simulink model "Charge_2_V1_FreeCharge"  (R2018b)
settings: Solver=FixedStepDiscrete  StartTime=0.0  StopTime=1  FixedStep=0.001  RelTol=1e-3
PreLoadFcn:
  | librarySetup
  | eval([bdroot,'_startup']) %Calling [modelName]_startup.m
undefined symbols (not defined in the file or in its folder): A0, A1, Car1__Authorize, Car2_Authorize, CON2, CON3, CON4, Control_Mode_In, CurrentSP, D10, D12, D13, D2, D3, D4, D5, D6, D7, D8, Free_Charge, Frequency_High_Point, Frequency_Low_Point, Frequency_Mid_high, Frequency_Mid_low, HVol_High_Point, HVol_Low_Point, HVol_Mid_high, HVol_Mid_low, HVoltage_Factor, SeconCar_ThreePhase, V_Current_five, V_Current_four, V_Current_one, V_Current_six, V_Current_three, V_Current_two, V_Frequency, V_MaxPliot, V_MinPliot, Vol_High_Point, Vol_Low_Point, Vol_Mid_high, Vol_Mid_low, Voltage_Factor, Voltage_Mode_Test
libraries: simulink x331, HANcoder_STM32_Target x30, powerlib_meascontrol x8, simulink_extras x2
(part 7 of 13)

== system Charge_2_V1_FreeCharge/HANcoder STM32 Target - E407-STM32 algorithm/Energy Meter1/Energy_Meter_Recieve/Voltage_Meter_2/Read_Gyro12 ==
  Trigger : TriggerPort  VariantControl=Variant
  UART receive : Subsystem  AncestorBlock=HANcoder_STM32_Target/STM32-E407/UART/UART receive  mask(UART receive){channel=UART2: Con. PD-8 & Con. PD-9 (PD5 & PD6), useStatusOut=off, tsamp=-1}
      mask prompts: useStatusOut "Use status outport"; tsamp "Sample time"
      mask help:
      | Function
      | ==========
      | Reads a byte from the UART reception buffer.
      |
      | Parameters per channel
      | ======================
      | - Select channel
      | - Select if the status output should be enabled.
      |
      | Outputs
      | =======
      | - The value of the receive byte.
      | - When the status output is 0, the reception buffer was empty.
      mask init:
      | uartChannelInfoStr = sfcn_uart_receive_mcb(2, channel, useStatusOut);
      settings: MoveFcn=drawLogos
      mask Help: web('sfcn_uart_receive.html')
      mask TypeOptions channel: UART1: Con. 3-D1 & Con. 3-D0 (PB6 & PB7) | UART2: Con. PD-8 & Con. PD-9 (PD5 & PD6) | UART3: Con. PD-11 & Con. PD-12 (PD8 & PD9) | UART6: Con. UEXT-3 & Con. UEXT-4 (PC6 & PC7)
      mask Display: fprintf('UART receive\n%s', uartChannelInfoStr);patch([240 246 246],[8 14 2],[1 0 0]);patch([248 248 254],[14 2 8],[0 0 0.35]);
  Out1 : Outport
  wires:
  UART receive/1(Out1) -> Out1/1

== system Charge_2_V1_FreeCharge/HANcoder STM32 Target - E407-STM32 algorithm/Energy Meter1/Energy_Meter_Recieve/Voltage_Meter_2/Read_Gyro13 ==
  Trigger : TriggerPort  VariantControl=Variant
  UART receive : Subsystem  AncestorBlock=HANcoder_STM32_Target/STM32-E407/UART/UART receive  mask(UART receive){channel=UART2: Con. PD-8 & Con. PD-9 (PD5 & PD6), useStatusOut=off, tsamp=-1}
      mask prompts: useStatusOut "Use status outport"; tsamp "Sample time"
      mask help:
      | Function
      | ==========
      | Reads a byte from the UART reception buffer.
      |
      | Parameters per channel
      | ======================
      | - Select channel
      | - Select if the status output should be enabled.
      |
      | Outputs
      | =======
      | - The value of the receive byte.
      | - When the status output is 0, the reception buffer was empty.
      mask init:
      | uartChannelInfoStr = sfcn_uart_receive_mcb(2, channel, useStatusOut);
      settings: MoveFcn=drawLogos
      mask Help: web('sfcn_uart_receive.html')
      mask TypeOptions channel: UART1: Con. 3-D1 & Con. 3-D0 (PB6 & PB7) | UART2: Con. PD-8 & Con. PD-9 (PD5 & PD6) | UART3: Con. PD-11 & Con. PD-12 (PD8 & PD9) | UART6: Con. UEXT-3 & Con. UEXT-4 (PC6 & PC7)
      mask Display: fprintf('UART receive\n%s', uartChannelInfoStr);patch([240 246 246],[8 14 2],[1 0 0]);patch([248 248 254],[14 2 8],[0 0 0.35]);
  Out1 : Outport
  wires:
  UART receive/1(Out1) -> Out1/1

== system Charge_2_V1_FreeCharge/HANcoder STM32 Target - E407-STM32 algorithm/Energy Meter1/Energy_Meter_Recieve/Voltage_Meter_2/Read_Gyro14 ==
  Trigger : TriggerPort  VariantControl=Variant
  UART receive : Subsystem  AncestorBlock=HANcoder_STM32_Target/STM32-E407/UART/UART receive  mask(UART receive){channel=UART2: Con. PD-8 & Con. PD-9 (PD5 & PD6), useStatusOut=off, tsamp=-1}
      mask prompts: useStatusOut "Use status outport"; tsamp "Sample time"
      mask help:
      | Function
      | ==========
      | Reads a byte from the UART reception buffer.
      |
      | Parameters per channel
      | ======================
      | - Select channel
      | - Select if the status output should be enabled.
      |
      | Outputs
      | =======
      | - The value of the receive byte.
      | - When the status output is 0, the reception buffer was empty.
      mask init:
      | uartChannelInfoStr = sfcn_uart_receive_mcb(2, channel, useStatusOut);
      settings: MoveFcn=drawLogos
      mask Help: web('sfcn_uart_receive.html')
      mask TypeOptions channel: UART1: Con. 3-D1 & Con. 3-D0 (PB6 & PB7) | UART2: Con. PD-8 & Con. PD-9 (PD5 & PD6) | UART3: Con. PD-11 & Con. PD-12 (PD8 & PD9) | UART6: Con. UEXT-3 & Con. UEXT-4 (PC6 & PC7)
      mask Display: fprintf('UART receive\n%s', uartChannelInfoStr);patch([240 246 246],[8 14 2],[1 0 0]);patch([248 248 254],[14 2 8],[0 0 0.35]);
  Out1 : Outport
  wires:
  UART receive/1(Out1) -> Out1/1

== system Charge_2_V1_FreeCharge/HANcoder STM32 Target - E407-STM32 algorithm/Energy Meter1/Energy_Meter_Recieve/Voltage_Meter_2/Read_Gyro15 ==
  Trigger : TriggerPort  VariantControl=Variant
  UART receive : Subsystem  AncestorBlock=HANcoder_STM32_Target/STM32-E407/UART/UART receive  mask(UART receive){channel=UART2: Con. PD-8 & Con. PD-9 (PD5 & PD6), useStatusOut=off, tsamp=-1}
      mask prompts: useStatusOut "Use status outport"; tsamp "Sample time"
      mask help:
      | Function
      | ==========
      | Reads a byte from the UART reception buffer.
      |
      | Parameters per channel
      | ======================
      | - Select channel
      | - Select if the status output should be enabled.
      |
      | Outputs
      | =======
      | - The value of the receive byte.
      | - When the status output is 0, the reception buffer was empty.
      mask init:
      | uartChannelInfoStr = sfcn_uart_receive_mcb(2, channel, useStatusOut);
      settings: MoveFcn=drawLogos
      mask Help: web('sfcn_uart_receive.html')
      mask TypeOptions channel: UART1: Con. 3-D1 & Con. 3-D0 (PB6 & PB7) | UART2: Con. PD-8 & Con. PD-9 (PD5 & PD6) | UART3: Con. PD-11 & Con. PD-12 (PD8 & PD9) | UART6: Con. UEXT-3 & Con. UEXT-4 (PC6 & PC7)
      mask Display: fprintf('UART receive\n%s', uartChannelInfoStr);patch([240 246 246],[8 14 2],[1 0 0]);patch([248 248 254],[14 2 8],[0 0 0.35]);
  Out1 : Outport
  wires:
  UART receive/1(Out1) -> Out1/1

== system Charge_2_V1_FreeCharge/HANcoder STM32 Target - E407-STM32 algorithm/Energy Meter1/Energy_Meter_Recieve/Voltage_Meter_2/Read_Gyro16 ==
  Trigger : TriggerPort  VariantControl=Variant
  UART receive : Subsystem  AncestorBlock=HANcoder_STM32_Target/STM32-E407/UART/UART receive  mask(UART receive){channel=UART2: Con. PD-8 & Con. PD-9 (PD5 & PD6), useStatusOut=off, tsamp=-1}
      mask prompts: useStatusOut "Use status outport"; tsamp "Sample time"
      mask help:
      | Function
      | ==========
      | Reads a byte from the UART reception buffer.
      |
      | Parameters per channel
      | ======================
      | - Select channel
      | - Select if the status output should be enabled.
      |
      | Outputs
      | =======
      | - The value of the receive byte.
      | - When the status output is 0, the reception buffer was empty.
      mask init:
      | uartChannelInfoStr = sfcn_uart_receive_mcb(2, channel, useStatusOut);
      settings: MoveFcn=drawLogos
      mask Help: web('sfcn_uart_receive.html')
      mask TypeOptions channel: UART1: Con. 3-D1 & Con. 3-D0 (PB6 & PB7) | UART2: Con. PD-8 & Con. PD-9 (PD5 & PD6) | UART3: Con. PD-11 & Con. PD-12 (PD8 & PD9) | UART6: Con. UEXT-3 & Con. UEXT-4 (PC6 & PC7)
      mask Display: fprintf('UART receive\n%s', uartChannelInfoStr);patch([240 246 246],[8 14 2],[1 0 0]);patch([248 248 254],[14 2 8],[0 0 0.35]);
  Out1 : Outport
  wires:
  UART receive/1(Out1) -> Out1/1

== system Charge_2_V1_FreeCharge/HANcoder STM32 Target - E407-STM32 algorithm/Energy Meter1/Energy_Meter_Recieve/Voltage_Meter_2/Read_Gyro17 ==
  Trigger : TriggerPort  VariantControl=Variant
  UART receive : Subsystem  AncestorBlock=HANcoder_STM32_Target/STM32-E407/UART/UART receive  mask(UART receive){channel=UART2: Con. PD-8 & Con. PD-9 (PD5 & PD6), useStatusOut=off, tsamp=-1}
      mask prompts: useStatusOut "Use status outport"; tsamp "Sample time"
      mask help:
      | Function
      | ==========
      | Reads a byte from the UART reception buffer.
      |
      | Parameters per channel
      | ======================
      | - Select channel
      | - Select if the status output should be enabled.
      |
      | Outputs
      | =======
      | - The value of the receive byte.
      | - When the status output is 0, the reception buffer was empty.
      mask init:
      | uartChannelInfoStr = sfcn_uart_receive_mcb(2, channel, useStatusOut);
      settings: MoveFcn=drawLogos
      mask Help: web('sfcn_uart_receive.html')
      mask TypeOptions channel: UART1: Con. 3-D1 & Con. 3-D0 (PB6 & PB7) | UART2: Con. PD-8 & Con. PD-9 (PD5 & PD6) | UART3: Con. PD-11 & Con. PD-12 (PD8 & PD9) | UART6: Con. UEXT-3 & Con. UEXT-4 (PC6 & PC7)
      mask Display: fprintf('UART receive\n%s', uartChannelInfoStr);patch([240 246 246],[8 14 2],[1 0 0]);patch([248 248 254],[14 2 8],[0 0 0.35]);
  Out1 : Outport
  wires:
  UART receive/1(Out1) -> Out1/1

== system Charge_2_V1_FreeCharge/HANcoder STM32 Target - E407-STM32 algorithm/Energy Meter1/Energy_Meter_Recieve/Voltage_Meter_2/Read_Gyro18 ==
  Trigger : TriggerPort  VariantControl=Variant
  UART receive : Subsystem  AncestorBlock=HANcoder_STM32_Target/STM32-E407/UART/UART receive  mask(UART receive){channel=UART2: Con. PD-8 & Con. PD-9 (PD5 & PD6), useStatusOut=off, tsamp=-1}
      mask prompts: useStatusOut "Use status outport"; tsamp "Sample time"
      mask help:
      | Function
      | ==========
      | Reads a byte from the UART reception buffer.
      |
      | Parameters per channel
      | ======================
      | - Select channel
      | - Select if the status output should be enabled.
      |
      | Outputs
      | =======
      | - The value of the receive byte.
      | - When the status output is 0, the reception buffer was empty.
      mask init:
      | uartChannelInfoStr = sfcn_uart_receive_mcb(2, channel, useStatusOut);
      settings: MoveFcn=drawLogos
      mask Help: web('sfcn_uart_receive.html')
      mask TypeOptions channel: UART1: Con. 3-D1 & Con. 3-D0 (PB6 & PB7) | UART2: Con. PD-8 & Con. PD-9 (PD5 & PD6) | UART3: Con. PD-11 & Con. PD-12 (PD8 & PD9) | UART6: Con. UEXT-3 & Con. UEXT-4 (PC6 & PC7)
      mask Display: fprintf('UART receive\n%s', uartChannelInfoStr);patch([240 246 246],[8 14 2],[1 0 0]);patch([248 248 254],[14 2 8],[0 0 0.35]);
  Out1 : Outport
  wires:
  UART receive/1(Out1) -> Out1/1

== system Charge_2_V1_FreeCharge/HANcoder STM32 Target - E407-STM32 algorithm/Energy Meter1/Energy_Meter_Recieve/Voltage_Meter_2/Read_Gyro2 ==
  Trigger : TriggerPort  VariantControl=Variant
  UART receive : Subsystem  AncestorBlock=HANcoder_STM32_Target/STM32-E407/UART/UART receive  mask(UART receive){channel=UART2: Con. PD-8 & Con. PD-9 (PD5 & PD6), useStatusOut=off, tsamp=-1}
      mask prompts: useStatusOut "Use status outport"; tsamp "Sample time"
      mask help:
      | Function
      | ==========
      | Reads a byte from the UART reception buffer.
      |
      | Parameters per channel
      | ======================
      | - Select channel
      | - Select if the status output should be enabled.
      |
      | Outputs
      | =======
      | - The value of the receive byte.
      | - When the status output is 0, the reception buffer was empty.
      mask init:
      | uartChannelInfoStr = sfcn_uart_receive_mcb(2, channel, useStatusOut);
      settings: MoveFcn=drawLogos
      mask Help: web('sfcn_uart_receive.html')
      mask TypeOptions channel: UART1: Con. 3-D1 & Con. 3-D0 (PB6 & PB7) | UART2: Con. PD-8 & Con. PD-9 (PD5 & PD6) | UART3: Con. PD-11 & Con. PD-12 (PD8 & PD9) | UART6: Con. UEXT-3 & Con. UEXT-4 (PC6 & PC7)
      mask Display: fprintf('UART receive\n%s', uartChannelInfoStr);patch([240 246 246],[8 14 2],[1 0 0]);patch([248 248 254],[14 2 8],[0 0 0.35]);
  Out1 : Outport
  wires:
  UART receive/1(Out1) -> Out1/1

== system Charge_2_V1_FreeCharge/HANcoder STM32 Target - E407-STM32 algorithm/Energy Meter1/Energy_Meter_Recieve/Voltage_Meter_2/Read_Gyro3 ==
  Trigger : TriggerPort  VariantControl=Variant
  UART receive : Subsystem  AncestorBlock=HANcoder_STM32_Target/STM32-E407/UART/UART receive  mask(UART receive){channel=UART2: Con. PD-8 & Con. PD-9 (PD5 & PD6), useStatusOut=off, tsamp=-1}
      mask prompts: useStatusOut "Use status outport"; tsamp "Sample time"
      mask help:
      | Function
      | ==========
      | Reads a byte from the UART reception buffer.
      |
      | Parameters per channel
      | ======================
      | - Select channel
      | - Select if the status output should be enabled.
      |
      | Outputs
      | =======
      | - The value of the receive byte.
      | - When the status output is 0, the reception buffer was empty.
      mask init:
      | uartChannelInfoStr = sfcn_uart_receive_mcb(2, channel, useStatusOut);
      settings: MoveFcn=drawLogos
      mask Help: web('sfcn_uart_receive.html')
      mask TypeOptions channel: UART1: Con. 3-D1 & Con. 3-D0 (PB6 & PB7) | UART2: Con. PD-8 & Con. PD-9 (PD5 & PD6) | UART3: Con. PD-11 & Con. PD-12 (PD8 & PD9) | UART6: Con. UEXT-3 & Con. UEXT-4 (PC6 & PC7)
      mask Display: fprintf('UART receive\n%s', uartChannelInfoStr);patch([240 246 246],[8 14 2],[1 0 0]);patch([248 248 254],[14 2 8],[0 0 0.35]);
  Out1 : Outport
  wires:
  UART receive/1(Out1) -> Out1/1

== system Charge_2_V1_FreeCharge/HANcoder STM32 Target - E407-STM32 algorithm/Energy Meter1/Energy_Meter_Recieve/Voltage_Meter_2/Read_Gyro4 ==
  Trigger : TriggerPort  VariantControl=Variant
  UART receive : Subsystem  AncestorBlock=HANcoder_STM32_Target/STM32-E407/UART/UART receive  mask(UART receive){channel=UART2: Con. PD-8 & Con. PD-9 (PD5 & PD6), useStatusOut=off, tsamp=-1}
      mask prompts: useStatusOut "Use status outport"; tsamp "Sample time"
      mask help:
      | Function
      | ==========
      | Reads a byte from the UART reception buffer.
      |
      | Parameters per channel
      | ======================
      | - Select channel
      | - Select if the status output should be enabled.
      |
      | Outputs
      | =======
      | - The value of the receive byte.
      | - When the status output is 0, the reception buffer was empty.
      mask init:
      | uartChannelInfoStr = sfcn_uart_receive_mcb(2, channel, useStatusOut);
      settings: MoveFcn=drawLogos
      mask Help: web('sfcn_uart_receive.html')
      mask TypeOptions channel: UART1: Con. 3-D1 & Con. 3-D0 (PB6 & PB7) | UART2: Con. PD-8 & Con. PD-9 (PD5 & PD6) | UART3: Con. PD-11 & Con. PD-12 (PD8 & PD9) | UART6: Con. UEXT-3 & Con. UEXT-4 (PC6 & PC7)
      mask Display: fprintf('UART receive\n%s', uartChannelInfoStr);patch([240 246 246],[8 14 2],[1 0 0]);patch([248 248 254],[14 2 8],[0 0 0.35]);
  Out1 : Outport
  wires:
  UART receive/1(Out1) -> Out1/1

== system Charge_2_V1_FreeCharge/HANcoder STM32 Target - E407-STM32 algorithm/Energy Meter1/Energy_Meter_Recieve/Voltage_Meter_2/Read_Gyro5 ==
  Trigger : TriggerPort  VariantControl=Variant
  UART receive : Subsystem  AncestorBlock=HANcoder_STM32_Target/STM32-E407/UART/UART receive  mask(UART receive){channel=UART2: Con. PD-8 & Con. PD-9 (PD5 & PD6), useStatusOut=off, tsamp=-1}
      mask prompts: useStatusOut "Use status outport"; tsamp "Sample time"
      mask help:
      | Function
      | ==========
      | Reads a byte from the UART reception buffer.
      |
      | Parameters per channel
      | ======================
      | - Select channel
      | - Select if the status output should be enabled.
      |
      | Outputs
      | =======
      | - The value of the receive byte.
      | - When the status output is 0, the reception buffer was empty.
      mask init:
      | uartChannelInfoStr = sfcn_uart_receive_mcb(2, channel, useStatusOut);
      settings: MoveFcn=drawLogos
      mask Help: web('sfcn_uart_receive.html')
      mask TypeOptions channel: UART1: Con. 3-D1 & Con. 3-D0 (PB6 & PB7) | UART2: Con. PD-8 & Con. PD-9 (PD5 & PD6) | UART3: Con. PD-11 & Con. PD-12 (PD8 & PD9) | UART6: Con. UEXT-3 & Con. UEXT-4 (PC6 & PC7)
      mask Display: fprintf('UART receive\n%s', uartChannelInfoStr);patch([240 246 246],[8 14 2],[1 0 0]);patch([248 248 254],[14 2 8],[0 0 0.35]);
  Out1 : Outport
  wires:
  UART receive/1(Out1) -> Out1/1

== system Charge_2_V1_FreeCharge/HANcoder STM32 Target - E407-STM32 algorithm/Energy Meter1/Energy_Meter_Recieve/Voltage_Meter_2/Read_Gyro6 ==
  Trigger : TriggerPort  VariantControl=Variant
  UART receive : Subsystem  AncestorBlock=HANcoder_STM32_Target/STM32-E407/UART/UART receive  mask(UART receive){channel=UART2: Con. PD-8 & Con. PD-9 (PD5 & PD6), useStatusOut=off, tsamp=-1}
      mask prompts: useStatusOut "Use status outport"; tsamp "Sample time"
      mask help:
      | Function
      | ==========
      | Reads a byte from the UART reception buffer.
      |
      | Parameters per channel
      | ======================
      | - Select channel
      | - Select if the status output should be enabled.
      |
      | Outputs
      | =======
      | - The value of the receive byte.
      | - When the status output is 0, the reception buffer was empty.
      mask init:
      | uartChannelInfoStr = sfcn_uart_receive_mcb(2, channel, useStatusOut);
      settings: MoveFcn=drawLogos
      mask Help: web('sfcn_uart_receive.html')
      mask TypeOptions channel: UART1: Con. 3-D1 & Con. 3-D0 (PB6 & PB7) | UART2: Con. PD-8 & Con. PD-9 (PD5 & PD6) | UART3: Con. PD-11 & Con. PD-12 (PD8 & PD9) | UART6: Con. UEXT-3 & Con. UEXT-4 (PC6 & PC7)
      mask Display: fprintf('UART receive\n%s', uartChannelInfoStr);patch([240 246 246],[8 14 2],[1 0 0]);patch([248 248 254],[14 2 8],[0 0 0.35]);
  Out1 : Outport
  wires:
  UART receive/1(Out1) -> Out1/1

== system Charge_2_V1_FreeCharge/HANcoder STM32 Target - E407-STM32 algorithm/Energy Meter1/Energy_Meter_Recieve/Voltage_Meter_2/Read_Gyro7 ==
  Trigger : TriggerPort  VariantControl=Variant
  UART receive : Subsystem  AncestorBlock=HANcoder_STM32_Target/STM32-E407/UART/UART receive  mask(UART receive){channel=UART2: Con. PD-8 & Con. PD-9 (PD5 & PD6), useStatusOut=off, tsamp=-1}
      mask prompts: useStatusOut "Use status outport"; tsamp "Sample time"
      mask help:
      | Function
      | ==========
      | Reads a byte from the UART reception buffer.
      |
      | Parameters per channel
      | ======================
      | - Select channel
      | - Select if the status output should be enabled.
      |
      | Outputs
      | =======
      | - The value of the receive byte.
      | - When the status output is 0, the reception buffer was empty.
      mask init:
      | uartChannelInfoStr = sfcn_uart_receive_mcb(2, channel, useStatusOut);
      settings: MoveFcn=drawLogos
      mask Help: web('sfcn_uart_receive.html')
      mask TypeOptions channel: UART1: Con. 3-D1 & Con. 3-D0 (PB6 & PB7) | UART2: Con. PD-8 & Con. PD-9 (PD5 & PD6) | UART3: Con. PD-11 & Con. PD-12 (PD8 & PD9) | UART6: Con. UEXT-3 & Con. UEXT-4 (PC6 & PC7)
      mask Display: fprintf('UART receive\n%s', uartChannelInfoStr);patch([240 246 246],[8 14 2],[1 0 0]);patch([248 248 254],[14 2 8],[0 0 0.35]);
  Out1 : Outport
  wires:
  UART receive/1(Out1) -> Out1/1

== system Charge_2_V1_FreeCharge/HANcoder STM32 Target - E407-STM32 algorithm/Energy Meter1/Energy_Meter_Recieve/Voltage_Meter_2/Read_Gyro8 ==
  Trigger : TriggerPort  VariantControl=Variant
  UART receive : Subsystem  AncestorBlock=HANcoder_STM32_Target/STM32-E407/UART/UART receive  mask(UART receive){channel=UART2: Con. PD-8 & Con. PD-9 (PD5 & PD6), useStatusOut=off, tsamp=-1}
      mask prompts: useStatusOut "Use status outport"; tsamp "Sample time"
      mask help:
      | Function
      | ==========
      | Reads a byte from the UART reception buffer.
      |
      | Parameters per channel
      | ======================
      | - Select channel
      | - Select if the status output should be enabled.
      |
      | Outputs
      | =======
      | - The value of the receive byte.
      | - When the status output is 0, the reception buffer was empty.
      mask init:
      | uartChannelInfoStr = sfcn_uart_receive_mcb(2, channel, useStatusOut);
      settings: MoveFcn=drawLogos
      mask Help: web('sfcn_uart_receive.html')
      mask TypeOptions channel: UART1: Con. 3-D1 & Con. 3-D0 (PB6 & PB7) | UART2: Con. PD-8 & Con. PD-9 (PD5 & PD6) | UART3: Con. PD-11 & Con. PD-12 (PD8 & PD9) | UART6: Con. UEXT-3 & Con. UEXT-4 (PC6 & PC7)
      mask Display: fprintf('UART receive\n%s', uartChannelInfoStr);patch([240 246 246],[8 14 2],[1 0 0]);patch([248 248 254],[14 2 8],[0 0 0.35]);
  Out1 : Outport
  wires:
  UART receive/1(Out1) -> Out1/1

== system Charge_2_V1_FreeCharge/HANcoder STM32 Target - E407-STM32 algorithm/Energy Meter1/Energy_Meter_Recieve/Voltage_Meter_2/Read_Gyro9 ==
  Trigger : TriggerPort  VariantControl=Variant
  UART receive : Subsystem  AncestorBlock=HANcoder_STM32_Target/STM32-E407/UART/UART receive  mask(UART receive){channel=UART2: Con. PD-8 & Con. PD-9 (PD5 & PD6), useStatusOut=off, tsamp=-1}
      mask prompts: useStatusOut "Use status outport"; tsamp "Sample time"
      mask help:
      | Function
      | ==========
      | Reads a byte from the UART reception buffer.
      |
      | Parameters per channel
      | ======================
      | - Select channel
      | - Select if the status output should be enabled.
      |
      | Outputs
      | =======
      | - The value of the receive byte.
      | - When the status output is 0, the reception buffer was empty.
      mask init:
      | uartChannelInfoStr = sfcn_uart_receive_mcb(2, channel, useStatusOut);
      settings: MoveFcn=drawLogos
      mask Help: web('sfcn_uart_receive.html')
      mask TypeOptions channel: UART1: Con. 3-D1 & Con. 3-D0 (PB6 & PB7) | UART2: Con. PD-8 & Con. PD-9 (PD5 & PD6) | UART3: Con. PD-11 & Con. PD-12 (PD8 & PD9) | UART6: Con. UEXT-3 & Con. UEXT-4 (PC6 & PC7)
      mask Display: fprintf('UART receive\n%s', uartChannelInfoStr);patch([240 246 246],[8 14 2],[1 0 0]);patch([248 248 254],[14 2 8],[0 0 0.35]);
  Out1 : Outport
  wires:
  UART receive/1(Out1) -> Out1/1

== system Charge_2_V1_FreeCharge/HANcoder STM32 Target - E407-STM32 algorithm/Energy Meter1/Energymeter_Request/Current_Meter_1 /Read_Gyro1 ==
  note: 01040000000271CB
  Trigger : TriggerPort  VariantControl=Variant
  Constant : Constant  Value=hex2dec('01')  OutDataTypeStr=uint8  SampleTime=-1
  UART send : Subsystem  Tag=HANcoder_TARGET_STM32_E407  AncestorBlock=HANcoder_STM32_Target/STM32-E407/UART/UART send  mask(UART send){channel=UART2: CON PD - 8 & 9, useStatusOut=off, tsamp=-1}
      mask prompts: useStatusOut "Use status outport"; tsamp "Sample time"
      mask help:
      | Function
      | ==========
      | Transmits a byte on the UART communication interface.
      |
      | Parameters per channel
      | ======================
      | - Select channel (TX & RX)
      | - Select if the status output should be enabled.
      |
      | Inputs
      | ======
      | - The byte to send
      |
      | Outputs
      | =======
      | - When the status output is 0, the byte could not be transmitted. Probably
      |   because the transmit buffer was configured too small.
      mask init:
      | uartChannelInfoStr = sfcn_uart_send_mcb(2, channel, useStatusOut);
      settings: MoveFcn=drawLogos
      mask Help: web('sfcn_uart_send.html')
      mask TypeOptions channel: UART1: CON3 - D1 & D0 | UART2: CON PD - 8 & 9 | UART3: CON PD - 11 & 12 | UART6: UEXT - 3 & 4
      mask Display: fprintf('UART send\n%s', uartChannelInfoStr);patch([245 251 251],[8 14 2],[1 0 0]);patch([253 253 259],[14 2 8],[0 0 0.35]);
  wires:
  Constant/1 -> UART send/1(In1)  "Sent_to_MCU"

== system Charge_2_V1_FreeCharge/HANcoder STM32 Target - E407-STM32 algorithm/Energy Meter1/Energymeter_Request/Current_Meter_1 /Read_Gyro2 ==
  note: 01040000000271CB
  Trigger : TriggerPort  VariantControl=Variant
  Constant1 : Constant  Value=hex2dec('04')  OutDataTypeStr=uint8  SampleTime=-1
  UART send : Subsystem  Tag=HANcoder_TARGET_STM32_E407  AncestorBlock=HANcoder_STM32_Target/STM32-E407/UART/UART send  mask(UART send){channel=UART2: CON PD - 8 & 9, useStatusOut=off, tsamp=-1}
      mask prompts: useStatusOut "Use status outport"; tsamp "Sample time"
      mask help:
      | Function
      | ==========
      | Transmits a byte on the UART communication interface.
      |
      | Parameters per channel
      | ======================
      | - Select channel (TX & RX)
      | - Select if the status output should be enabled.
      |
      | Inputs
      | ======
      | - The byte to send
      |
      | Outputs
      | =======
      | - When the status output is 0, the byte could not be transmitted. Probably
      |   because the transmit buffer was configured too small.
      mask init:
      | uartChannelInfoStr = sfcn_uart_send_mcb(2, channel, useStatusOut);
      settings: MoveFcn=drawLogos
      mask Help: web('sfcn_uart_send.html')
      mask TypeOptions channel: UART1: CON3 - D1 & D0 | UART2: CON PD - 8 & 9 | UART3: CON PD - 11 & 12 | UART6: UEXT - 3 & 4
      mask Display: fprintf('UART send\n%s', uartChannelInfoStr);patch([245 251 251],[8 14 2],[1 0 0]);patch([253 253 259],[14 2 8],[0 0 0.35]);
  wires:
  Constant1/1 -> UART send/1(In1)

== system Charge_2_V1_FreeCharge/HANcoder STM32 Target - E407-STM32 algorithm/Energy Meter1/Energymeter_Request/Current_Meter_1 /Read_Gyro3 ==
  note: 01040000000271CB
  Trigger : TriggerPort  VariantControl=Variant
  Constant2 : Constant  Value=hex2dec('00')  OutDataTypeStr=uint8  SampleTime=-1
  UART send : Subsystem  Tag=HANcoder_TARGET_STM32_E407  AncestorBlock=HANcoder_STM32_Target/STM32-E407/UART/UART send  mask(UART send){channel=UART2: CON PD - 8 & 9, useStatusOut=off, tsamp=-1}
      mask prompts: useStatusOut "Use status outport"; tsamp "Sample time"
      mask help:
      | Function
      | ==========
      | Transmits a byte on the UART communication interface.
      |
      | Parameters per channel
      | ======================
      | - Select channel (TX & RX)
      | - Select if the status output should be enabled.
      |
      | Inputs
      | ======
      | - The byte to send
      |
      | Outputs
      | =======
      | - When the status output is 0, the byte could not be transmitted. Probably
      |   because the transmit buffer was configured too small.
      mask init:
      | uartChannelInfoStr = sfcn_uart_send_mcb(2, channel, useStatusOut);
      settings: MoveFcn=drawLogos
      mask Help: web('sfcn_uart_send.html')
      mask TypeOptions channel: UART1: CON3 - D1 & D0 | UART2: CON PD - 8 & 9 | UART3: CON PD - 11 & 12 | UART6: UEXT - 3 & 4
      mask Display: fprintf('UART send\n%s', uartChannelInfoStr);patch([245 251 251],[8 14 2],[1 0 0]);patch([253 253 259],[14 2 8],[0 0 0.35]);
  wires:
  Constant2/1 -> UART send/1(In1)

== system Charge_2_V1_FreeCharge/HANcoder STM32 Target - E407-STM32 algorithm/Energy Meter1/Energymeter_Request/Current_Meter_1 /Read_Gyro4 ==
  note: 01040000000271CB
  Trigger : TriggerPort  VariantControl=Variant
  Constant4 : Constant  Value=hex2dec('6')  OutDataTypeStr=uint8  SampleTime=-1
  UART send : Subsystem  Tag=HANcoder_TARGET_STM32_E407  AncestorBlock=HANcoder_STM32_Target/STM32-E407/UART/UART send  mask(UART send){channel=UART2: CON PD - 8 & 9, useStatusOut=off, tsamp=-1}
      mask prompts: useStatusOut "Use status outport"; tsamp "Sample time"
      mask help:
      | Function
      | ==========
      | Transmits a byte on the UART communication interface.
      |
      | Parameters per channel
      | ======================
      | - Select channel (TX & RX)
      | - Select if the status output should be enabled.
      |
      | Inputs
      | ======
      | - The byte to send
      |
      | Outputs
      | =======
      | - When the status output is 0, the byte could not be transmitted. Probably
      |   because the transmit buffer was configured too small.
      mask init:
      | uartChannelInfoStr = sfcn_uart_send_mcb(2, channel, useStatusOut);
      settings: MoveFcn=drawLogos
      mask Help: web('sfcn_uart_send.html')
      mask TypeOptions channel: UART1: CON3 - D1 & D0 | UART2: CON PD - 8 & 9 | UART3: CON PD - 11 & 12 | UART6: UEXT - 3 & 4
      mask Display: fprintf('UART send\n%s', uartChannelInfoStr);patch([245 251 251],[8 14 2],[1 0 0]);patch([253 253 259],[14 2 8],[0 0 0.35]);
  wires:
  Constant4/1 -> UART send/1(In1)

== system Charge_2_V1_FreeCharge/HANcoder STM32 Target - E407-STM32 algorithm/Energy Meter1/Energymeter_Request/Current_Meter_1 /Read_Gyro5 ==
  note: 01040000000271CB
  Trigger : TriggerPort  VariantControl=Variant
  Constant5 : Constant  Value=hex2dec('00')  OutDataTypeStr=uint8  SampleTime=-1
  UART send : Subsystem  Tag=HANcoder_TARGET_STM32_E407  AncestorBlock=HANcoder_STM32_Target/STM32-E407/UART/UART send  mask(UART send){channel=UART2: CON PD - 8 & 9, useStatusOut=off, tsamp=-1}
      mask prompts: useStatusOut "Use status outport"; tsamp "Sample time"
      mask help:
      | Function
      | ==========
      | Transmits a byte on the UART communication interface.
      |
      | Parameters per channel
      | ======================
      | - Select channel (TX & RX)
      | - Select if the status output should be enabled.
      |
      | Inputs
      | ======
      | - The byte to send
      |
      | Outputs
      | =======
      | - When the status output is 0, the byte could not be transmitted. Probably
      |   because the transmit buffer was configured too small.
      mask init:
      | uartChannelInfoStr = sfcn_uart_send_mcb(2, channel, useStatusOut);
      settings: MoveFcn=drawLogos
      mask Help: web('sfcn_uart_send.html')
      mask TypeOptions channel: UART1: CON3 - D1 & D0 | UART2: CON PD - 8 & 9 | UART3: CON PD - 11 & 12 | UART6: UEXT - 3 & 4
      mask Display: fprintf('UART send\n%s', uartChannelInfoStr);patch([245 251 251],[8 14 2],[1 0 0]);patch([253 253 259],[14 2 8],[0 0 0.35]);
  wires:
  Constant5/1 -> UART send/1(In1)

== system Charge_2_V1_FreeCharge/HANcoder STM32 Target - E407-STM32 algorithm/Energy Meter1/Energymeter_Request/Current_Meter_1 /Read_Gyro6 ==
  note: 01040000000271CB
  Trigger : TriggerPort  VariantControl=Variant
  Constant6 : Constant  Value=hex2dec('06')  OutDataTypeStr=uint8  SampleTime=-1
  Terminator2 : Terminator
  UART send : Subsystem  Tag=HANcoder_TARGET_STM32_E407  AncestorBlock=HANcoder_STM32_Target/STM32-E407/UART/UART send  mask(UART send){channel=UART2: CON PD - 8 & 9, useStatusOut=off, tsamp=-1}
      mask prompts: useStatusOut "Use status outport"; tsamp "Sample time"
      mask help:
      | Function
      | ==========
      | Transmits a byte on the UART communication interface.
      |
      | Parameters per channel
      | ======================
      | - Select channel (TX & RX)
      | - Select if the status output should be enabled.
      |
      | Inputs
      | ======
      | - The byte to send
      |
      | Outputs
      | =======
      | - When the status output is 0, the byte could not be transmitted. Probably
      |   because the transmit buffer was configured too small.
      mask init:
      | uartChannelInfoStr = sfcn_uart_send_mcb(2, channel, useStatusOut);
      settings: MoveFcn=drawLogos
      mask Help: web('sfcn_uart_send.html')
      mask TypeOptions channel: UART1: CON3 - D1 & D0 | UART2: CON PD - 8 & 9 | UART3: CON PD - 11 & 12 | UART6: UEXT - 3 & 4
      mask Display: fprintf('UART send\n%s', uartChannelInfoStr);patch([245 251 251],[8 14 2],[1 0 0]);patch([253 253 259],[14 2 8],[0 0 0.35]);
  wires:
  Constant6/1 -> UART send/1(In1)

== system Charge_2_V1_FreeCharge/HANcoder STM32 Target - E407-STM32 algorithm/Energy Meter1/Energymeter_Request/Current_Meter_1 /Read_Gyro7 ==
  note: 01040000000271CB
  Trigger : TriggerPort  VariantControl=Variant
  Constant1 : Constant  Value=hex2dec('71')  OutDataTypeStr=uint8  SampleTime=-1
  Constant3 : Constant  Value=hex2dec('90')  OutDataTypeStr=uint8  SampleTime=-1
  UART send : Subsystem  Tag=HANcoder_TARGET_STM32_E407  AncestorBlock=HANcoder_STM32_Target/STM32-E407/UART/UART send  mask(UART send){channel=UART2: CON PD - 8 & 9, useStatusOut=off, tsamp=-1}
      mask prompts: useStatusOut "Use status outport"; tsamp "Sample time"
      mask help:
      | Function
      | ==========
      | Transmits a byte on the UART communication interface.
      |
      | Parameters per channel
      | ======================
      | - Select channel (TX & RX)
      | - Select if the status output should be enabled.
      |
      | Inputs
      | ======
      | - The byte to send
      |
      | Outputs
      | =======
      | - When the status output is 0, the byte could not be transmitted. Probably
      |   because the transmit buffer was configured too small.
      mask init:
      | uartChannelInfoStr = sfcn_uart_send_mcb(2, channel, useStatusOut);
      settings: MoveFcn=drawLogos
      mask Help: web('sfcn_uart_send.html')
      mask TypeOptions channel: UART1: CON3 - D1 & D0 | UART2: CON PD - 8 & 9 | UART3: CON PD - 11 & 12 | UART6: UEXT - 3 & 4
      mask Display: fprintf('UART send\n%s', uartChannelInfoStr);patch([245 251 251],[8 14 2],[1 0 0]);patch([253 253 259],[14 2 8],[0 0 0.35]);
  wires:
  Constant3/1 -> UART send/1(In1)

== system Charge_2_V1_FreeCharge/HANcoder STM32 Target - E407-STM32 algorithm/Energy Meter1/Energymeter_Request/Current_Meter_1 /Read_Gyro8 ==
  note: 01040000000271CB
  Trigger : TriggerPort  VariantControl=Variant
  Constant1 : Constant  Value=hex2dec('CB')  OutDataTypeStr=uint8  SampleTime=-1
  Constant7 : Constant  Value=hex2dec('09')  OutDataTypeStr=uint8  SampleTime=-1
  UART send : Subsystem  Tag=HANcoder_TARGET_STM32_E407  AncestorBlock=HANcoder_STM32_Target/STM32-E407/UART/UART send  mask(UART send){channel=UART2: CON PD - 8 & 9, useStatusOut=off, tsamp=-1}
      mask prompts: useStatusOut "Use status outport"; tsamp "Sample time"
      mask help:
      | Function
      | ==========
      | Transmits a byte on the UART communication interface.
      |
      | Parameters per channel
      | ======================
      | - Select channel (TX & RX)
      | - Select if the status output should be enabled.
      |
      | Inputs
      | ======
      | - The byte to send
      |
      | Outputs
      | =======
      | - When the status output is 0, the byte could not be transmitted. Probably
      |   because the transmit buffer was configured too small.
      mask init:
      | uartChannelInfoStr = sfcn_uart_send_mcb(2, channel, useStatusOut);
      settings: MoveFcn=drawLogos
      mask Help: web('sfcn_uart_send.html')
      mask TypeOptions channel: UART1: CON3 - D1 & D0 | UART2: CON PD - 8 & 9 | UART3: CON PD - 11 & 12 | UART6: UEXT - 3 & 4
      mask Display: fprintf('UART send\n%s', uartChannelInfoStr);patch([245 251 251],[8 14 2],[1 0 0]);patch([253 253 259],[14 2 8],[0 0 0.35]);
  wires:
  Constant7/1 -> UART send/1(In1)

== system Charge_2_V1_FreeCharge/HANcoder STM32 Target - E407-STM32 algorithm/Energy Meter1/Energymeter_Request/Current_Meter_2/Read_Gyro10 ==
  note: 01040000000271CB
  Trigger : TriggerPort  VariantControl=Variant
  Constant1 : Constant  Value=hex2dec('04')  OutDataTypeStr=uint8  SampleTime=-1
  UART send : Subsystem  Tag=HANcoder_TARGET_STM32_E407  AncestorBlock=HANcoder_STM32_Target/STM32-E407/UART/UART send  mask(UART send){channel=UART2: CON PD - 8 & 9, useStatusOut=off, tsamp=-1}
      mask prompts: useStatusOut "Use status outport"; tsamp "Sample time"
      mask help:
      | Function
      | ==========
      | Transmits a byte on the UART communication interface.
      |
      | Parameters per channel
      | ======================
      | - Select channel (TX & RX)
      | - Select if the status output should be enabled.
      |
      | Inputs
      | ======
      | - The byte to send
      |
      | Outputs
      | =======
      | - When the status output is 0, the byte could not be transmitted. Probably
      |   because the transmit buffer was configured too small.
      mask init:
      | uartChannelInfoStr = sfcn_uart_send_mcb(2, channel, useStatusOut);
      settings: MoveFcn=drawLogos
      mask Help: web('sfcn_uart_send.html')
      mask TypeOptions channel: UART1: CON3 - D1 & D0 | UART2: CON PD - 8 & 9 | UART3: CON PD - 11 & 12 | UART6: UEXT - 3 & 4
      mask Display: fprintf('UART send\n%s', uartChannelInfoStr);patch([245 251 251],[8 14 2],[1 0 0]);patch([253 253 259],[14 2 8],[0 0 0.35]);
  wires:
  Constant1/1 -> UART send/1(In1)

== system Charge_2_V1_FreeCharge/HANcoder STM32 Target - E407-STM32 algorithm/Energy Meter1/Energymeter_Request/Current_Meter_2/Read_Gyro11 ==
  note: 01040000000271CB
  Trigger : TriggerPort  VariantControl=Variant
  Constant2 : Constant  Value=hex2dec('00')  OutDataTypeStr=uint8  SampleTime=-1
  UART send : Subsystem  Tag=HANcoder_TARGET_STM32_E407  AncestorBlock=HANcoder_STM32_Target/STM32-E407/UART/UART send  mask(UART send){channel=UART2: CON PD - 8 & 9, useStatusOut=off, tsamp=-1}
      mask prompts: useStatusOut "Use status outport"; tsamp "Sample time"
      mask help:
      | Function
      | ==========
      | Transmits a byte on the UART communication interface.
      |
      | Parameters per channel
      | ======================
      | - Select channel (TX & RX)
      | - Select if the status output should be enabled.
      |
      | Inputs
      | ======
      | - The byte to send
      |
      | Outputs
      | =======
      | - When the status output is 0, the byte could not be transmitted. Probably
      |   because the transmit buffer was configured too small.
      mask init:
      | uartChannelInfoStr = sfcn_uart_send_mcb(2, channel, useStatusOut);
      settings: MoveFcn=drawLogos
      mask Help: web('sfcn_uart_send.html')
      mask TypeOptions channel: UART1: CON3 - D1 & D0 | UART2: CON PD - 8 & 9 | UART3: CON PD - 11 & 12 | UART6: UEXT - 3 & 4
      mask Display: fprintf('UART send\n%s', uartChannelInfoStr);patch([245 251 251],[8 14 2],[1 0 0]);patch([253 253 259],[14 2 8],[0 0 0.35]);
  wires:
  Constant2/1 -> UART send/1(In1)

== system Charge_2_V1_FreeCharge/HANcoder STM32 Target - E407-STM32 algorithm/Energy Meter1/Energymeter_Request/Current_Meter_2/Read_Gyro12 ==
  note: 01040000000271CB
  Trigger : TriggerPort  VariantControl=Variant
  Constant4 : Constant  Value=hex2dec('06')  OutDataTypeStr=uint8  SampleTime=-1
  UART send : Subsystem  Tag=HANcoder_TARGET_STM32_E407  AncestorBlock=HANcoder_STM32_Target/STM32-E407/UART/UART send  mask(UART send){channel=UART2: CON PD - 8 & 9, useStatusOut=off, tsamp=-1}
      mask prompts: useStatusOut "Use status outport"; tsamp "Sample time"
      mask help:
      | Function
      | ==========
      | Transmits a byte on the UART communication interface.
      |
      | Parameters per channel
      | ======================
      | - Select channel (TX & RX)
      | - Select if the status output should be enabled.
      |
      | Inputs
      | ======
      | - The byte to send
      |
      | Outputs
      | =======
      | - When the status output is 0, the byte could not be transmitted. Probably
      |   because the transmit buffer was configured too small.
      mask init:
      | uartChannelInfoStr = sfcn_uart_send_mcb(2, channel, useStatusOut);
      settings: MoveFcn=drawLogos
      mask Help: web('sfcn_uart_send.html')
      mask TypeOptions channel: UART1: CON3 - D1 & D0 | UART2: CON PD - 8 & 9 | UART3: CON PD - 11 & 12 | UART6: UEXT - 3 & 4
      mask Display: fprintf('UART send\n%s', uartChannelInfoStr);patch([245 251 251],[8 14 2],[1 0 0]);patch([253 253 259],[14 2 8],[0 0 0.35]);
  wires:
  Constant4/1 -> UART send/1(In1)

== system Charge_2_V1_FreeCharge/HANcoder STM32 Target - E407-STM32 algorithm/Energy Meter1/Energymeter_Request/Current_Meter_2/Read_Gyro13 ==
  note: 01040000000271CB
  Trigger : TriggerPort  VariantControl=Variant
  Constant5 : Constant  Value=hex2dec('00')  OutDataTypeStr=uint8  SampleTime=-1
  UART send : Subsystem  Tag=HANcoder_TARGET_STM32_E407  AncestorBlock=HANcoder_STM32_Target/STM32-E407/UART/UART send  mask(UART send){channel=UART2: CON PD - 8 & 9, useStatusOut=off, tsamp=-1}
      mask prompts: useStatusOut "Use status outport"; tsamp "Sample time"
      mask help:
      | Function
      | ==========
      | Transmits a byte on the UART communication interface.
      |
      | Parameters per channel
      | ======================
      | - Select channel (TX & RX)
      | - Select if the status output should be enabled.
      |
      | Inputs
      | ======
      | - The byte to send
      |
      | Outputs
      | =======
      | - When the status output is 0, the byte could not be transmitted. Probably
      |   because the transmit buffer was configured too small.
      mask init:
      | uartChannelInfoStr = sfcn_uart_send_mcb(2, channel, useStatusOut);
      settings: MoveFcn=drawLogos
      mask Help: web('sfcn_uart_send.html')
      mask TypeOptions channel: UART1: CON3 - D1 & D0 | UART2: CON PD - 8 & 9 | UART3: CON PD - 11 & 12 | UART6: UEXT - 3 & 4
      mask Display: fprintf('UART send\n%s', uartChannelInfoStr);patch([245 251 251],[8 14 2],[1 0 0]);patch([253 253 259],[14 2 8],[0 0 0.35]);
  wires:
  Constant5/1 -> UART send/1(In1)

== system Charge_2_V1_FreeCharge/HANcoder STM32 Target - E407-STM32 algorithm/Energy Meter1/Energymeter_Request/Current_Meter_2/Read_Gyro14 ==
  note: 01040000000271CB
  Trigger : TriggerPort  VariantControl=Variant
  Constant6 : Constant  Value=hex2dec('06')  OutDataTypeStr=uint8  SampleTime=-1
  Terminator2 : Terminator
  UART send : Subsystem  Tag=HANcoder_TARGET_STM32_E407  AncestorBlock=HANcoder_STM32_Target/STM32-E407/UART/UART send  mask(UART send){channel=UART2: CON PD - 8 & 9, useStatusOut=off, tsamp=-1}
      mask prompts: useStatusOut "Use status outport"; tsamp "Sample time"
      mask help:
      | Function
      | ==========
      | Transmits a byte on the UART communication interface.
      |
      | Parameters per channel
      | ======================
      | - Select channel (TX & RX)
      | - Select if the status output should be enabled.
      |
      | Inputs
      | ======
      | - The byte to send
      |
      | Outputs
      | =======
      | - When the status output is 0, the byte could not be transmitted. Probably
      |   because the transmit buffer was configured too small.
      mask init:
      | uartChannelInfoStr = sfcn_uart_send_mcb(2, channel, useStatusOut);
      settings: MoveFcn=drawLogos
      mask Help: web('sfcn_uart_send.html')
      mask TypeOptions channel: UART1: CON3 - D1 & D0 | UART2: CON PD - 8 & 9 | UART3: CON PD - 11 & 12 | UART6: UEXT - 3 & 4
      mask Display: fprintf('UART send\n%s', uartChannelInfoStr);patch([245 251 251],[8 14 2],[1 0 0]);patch([253 253 259],[14 2 8],[0 0 0.35]);
  wires:
  Constant6/1 -> UART send/1(In1)

== system Charge_2_V1_FreeCharge/HANcoder STM32 Target - E407-STM32 algorithm/Energy Meter1/Energymeter_Request/Current_Meter_2/Read_Gyro15 ==
  note: 01040000000271CB
  Trigger : TriggerPort  VariantControl=Variant
  Constant1 : Constant  Value=hex2dec('90')  OutDataTypeStr=uint8  SampleTime=-1
  UART send : Subsystem  Tag=HANcoder_TARGET_STM32_E407  AncestorBlock=HANcoder_STM32_Target/STM32-E407/UART/UART send  mask(UART send){channel=UART2: CON PD - 8 & 9, useStatusOut=off, tsamp=-1}
      mask prompts: useStatusOut "Use status outport"; tsamp "Sample time"
      mask help:
      | Function
      | ==========
      | Transmits a byte on the UART communication interface.
      |
      | Parameters per channel
      | ======================
      | - Select channel (TX & RX)
      | - Select if the status output should be enabled.
      |
      | Inputs
      | ======
      | - The byte to send
      |
      | Outputs
      | =======
      | - When the status output is 0, the byte could not be transmitted. Probably
      |   because the transmit buffer was configured too small.
      mask init:
      | uartChannelInfoStr = sfcn_uart_send_mcb(2, channel, useStatusOut);
      settings: MoveFcn=drawLogos
      mask Help: web('sfcn_uart_send.html')
      mask TypeOptions channel: UART1: CON3 - D1 & D0 | UART2: CON PD - 8 & 9 | UART3: CON PD - 11 & 12 | UART6: UEXT - 3 & 4
      mask Display: fprintf('UART send\n%s', uartChannelInfoStr);patch([245 251 251],[8 14 2],[1 0 0]);patch([253 253 259],[14 2 8],[0 0 0.35]);
  wires:
  Constant1/1 -> UART send/1(In1)

== system Charge_2_V1_FreeCharge/HANcoder STM32 Target - E407-STM32 algorithm/Energy Meter1/Energymeter_Request/Current_Meter_2/Read_Gyro16 ==
  note: 01040000000271CB
  Trigger : TriggerPort  VariantControl=Variant
  Constant1 : Constant  Value=hex2dec('3A')  OutDataTypeStr=uint8  SampleTime=-1
  UART send : Subsystem  Tag=HANcoder_TARGET_STM32_E407  AncestorBlock=HANcoder_STM32_Target/STM32-E407/UART/UART send  mask(UART send){channel=UART2: CON PD - 8 & 9, useStatusOut=off, tsamp=-1}
      mask prompts: useStatusOut "Use status outport"; tsamp "Sample time"
      mask help:
      | Function
      | ==========
      | Transmits a byte on the UART communication interface.
      |
      | Parameters per channel
      | ======================
      | - Select channel (TX & RX)
      | - Select if the status output should be enabled.
      |
      | Inputs
      | ======
      | - The byte to send
      |
      | Outputs
      | =======
      | - When the status output is 0, the byte could not be transmitted. Probably
      |   because the transmit buffer was configured too small.
      mask init:
      | uartChannelInfoStr = sfcn_uart_send_mcb(2, channel, useStatusOut);
      settings: MoveFcn=drawLogos
      mask Help: web('sfcn_uart_send.html')
      mask TypeOptions channel: UART1: CON3 - D1 & D0 | UART2: CON PD - 8 & 9 | UART3: CON PD - 11 & 12 | UART6: UEXT - 3 & 4
      mask Display: fprintf('UART send\n%s', uartChannelInfoStr);patch([245 251 251],[8 14 2],[1 0 0]);patch([253 253 259],[14 2 8],[0 0 0.35]);
  wires:
  Constant1/1 -> UART send/1(In1)

== system Charge_2_V1_FreeCharge/HANcoder STM32 Target - E407-STM32 algorithm/Energy Meter1/Energymeter_Request/Current_Meter_2/Read_Gyro9 ==
  note: 01040000000271CB
  Trigger : TriggerPort  VariantControl=Variant
  Constant : Constant  Value=hex2dec('02')  OutDataTypeStr=uint8  SampleTime=-1
  UART send : Subsystem  Tag=HANcoder_TARGET_STM32_E407  AncestorBlock=HANcoder_STM32_Target/STM32-E407/UART/UART send  mask(UART send){channel=UART2: CON PD - 8 & 9, useStatusOut=off, tsamp=-1}
      mask prompts: useStatusOut "Use status outport"; tsamp "Sample time"
      mask help:
      | Function
      | ==========
      | Transmits a byte on the UART communication interface.
      |
      | Parameters per channel
      | ======================
      | - Select channel (TX & RX)
      | - Select if the status output should be enabled.
      |
      | Inputs
      | ======
      | - The byte to send
      |
      | Outputs
      | =======
      | - When the status output is 0, the byte could not be transmitted. Probably
      |   because the transmit buffer was configured too small.
      mask init:
      | uartChannelInfoStr = sfcn_uart_send_mcb(2, channel, useStatusOut);
      settings: MoveFcn=drawLogos
      mask Help: web('sfcn_uart_send.html')
      mask TypeOptions channel: UART1: CON3 - D1 & D0 | UART2: CON PD - 8 & 9 | UART3: CON PD - 11 & 12 | UART6: UEXT - 3 & 4
      mask Display: fprintf('UART send\n%s', uartChannelInfoStr);patch([245 251 251],[8 14 2],[1 0 0]);patch([253 253 259],[14 2 8],[0 0 0.35]);
  wires:
  Constant/1 -> UART send/1(In1)

== system Charge_2_V1_FreeCharge/HANcoder STM32 Target - E407-STM32 algorithm/Energy Meter1/Energymeter_Request/Fequency/Read_Gyro10 ==
  note: 01040000000271CB
  Trigger : TriggerPort  VariantControl=Variant
  Constant1 : Constant  Value=hex2dec('04')  OutDataTypeStr=uint8  SampleTime=-1
  UART send : Subsystem  Tag=HANcoder_TARGET_STM32_E407  AncestorBlock=HANcoder_STM32_Target/STM32-E407/UART/UART send  mask(UART send){channel=UART2: CON PD - 8 & 9, useStatusOut=off, tsamp=-1}
      mask prompts: useStatusOut "Use status outport"; tsamp "Sample time"
      mask help:
      | Function
      | ==========
      | Transmits a byte on the UART communication interface.
      |
      | Parameters per channel
      | ======================
      | - Select channel (TX & RX)
      | - Select if the status output should be enabled.
      |
      | Inputs
      | ======
      | - The byte to send
      |
      | Outputs
      | =======
      | - When the status output is 0, the byte could not be transmitted. Probably
      |   because the transmit buffer was configured too small.
      mask init:
      | uartChannelInfoStr = sfcn_uart_send_mcb(2, channel, useStatusOut);
      settings: MoveFcn=drawLogos
      mask Help: web('sfcn_uart_send.html')
      mask TypeOptions channel: UART1: CON3 - D1 & D0 | UART2: CON PD - 8 & 9 | UART3: CON PD - 11 & 12 | UART6: UEXT - 3 & 4
      mask Display: fprintf('UART send\n%s', uartChannelInfoStr);patch([245 251 251],[8 14 2],[1 0 0]);patch([253 253 259],[14 2 8],[0 0 0.35]);
  wires:
  Constant1/1 -> UART send/1(In1)

== system Charge_2_V1_FreeCharge/HANcoder STM32 Target - E407-STM32 algorithm/Energy Meter1/Energymeter_Request/Fequency/Read_Gyro11 ==
  note: 01040000000271CB
  Trigger : TriggerPort  VariantControl=Variant
  Constant2 : Constant  Value=hex2dec('00')  OutDataTypeStr=uint8  SampleTime=-1
  UART send : Subsystem  Tag=HANcoder_TARGET_STM32_E407  AncestorBlock=HANcoder_STM32_Target/STM32-E407/UART/UART send  mask(UART send){channel=UART2: CON PD - 8 & 9, useStatusOut=off, tsamp=-1}
      mask prompts: useStatusOut "Use status outport"; tsamp "Sample time"
      mask help:
      | Function
      | ==========
      | Transmits a byte on the UART communication interface.
      |
      | Parameters per channel
      | ======================
      | - Select channel (TX & RX)
      | - Select if the status output should be enabled.
      |
      | Inputs
      | ======
      | - The byte to send
      |
      | Outputs
      | =======
      | - When the status output is 0, the byte could not be transmitted. Probably
      |   because the transmit buffer was configured too small.
      mask init:
      | uartChannelInfoStr = sfcn_uart_send_mcb(2, channel, useStatusOut);
      settings: MoveFcn=drawLogos
      mask Help: web('sfcn_uart_send.html')
      mask TypeOptions channel: UART1: CON3 - D1 & D0 | UART2: CON PD - 8 & 9 | UART3: CON PD - 11 & 12 | UART6: UEXT - 3 & 4
      mask Display: fprintf('UART send\n%s', uartChannelInfoStr);patch([245 251 251],[8 14 2],[1 0 0]);patch([253 253 259],[14 2 8],[0 0 0.35]);
  wires:
  Constant2/1 -> UART send/1(In1)

== system Charge_2_V1_FreeCharge/HANcoder STM32 Target - E407-STM32 algorithm/Energy Meter1/Energymeter_Request/Fequency/Read_Gyro12 ==
  note: 01040000000271CB
  Trigger : TriggerPort  VariantControl=Variant
  Constant4 : Constant  Value=hex2dec('46')  OutDataTypeStr=uint8  SampleTime=-1
  UART send : Subsystem  Tag=HANcoder_TARGET_STM32_E407  AncestorBlock=HANcoder_STM32_Target/STM32-E407/UART/UART send  mask(UART send){channel=UART2: CON PD - 8 & 9, useStatusOut=off, tsamp=-1}
      mask prompts: useStatusOut "Use status outport"; tsamp "Sample time"
      mask help:
      | Function
      | ==========
      | Transmits a byte on the UART communication interface.
      |
      | Parameters per channel
      | ======================
      | - Select channel (TX & RX)
      | - Select if the status output should be enabled.
      |
      | Inputs
      | ======
      | - The byte to send
      |
      | Outputs
      | =======
      | - When the status output is 0, the byte could not be transmitted. Probably
      |   because the transmit buffer was configured too small.
      mask init:
      | uartChannelInfoStr = sfcn_uart_send_mcb(2, channel, useStatusOut);
      settings: MoveFcn=drawLogos
      mask Help: web('sfcn_uart_send.html')
      mask TypeOptions channel: UART1: CON3 - D1 & D0 | UART2: CON PD - 8 & 9 | UART3: CON PD - 11 & 12 | UART6: UEXT - 3 & 4
      mask Display: fprintf('UART send\n%s', uartChannelInfoStr);patch([245 251 251],[8 14 2],[1 0 0]);patch([253 253 259],[14 2 8],[0 0 0.35]);
  wires:
  Constant4/1 -> UART send/1(In1)
